simulink model "B20_ATMD_Earthquake"  (R2020b)
settings: Solver=ode45  StartTime=0.0  StopTime=40  FixedStep=Ts  MaxStep=Ts  MinStep=0.005  RelTol=1e-2
values from neighbouring files (symbols this model uses):
  DoS_on = 0    [tuneCusum_Detector1.m]    (also in tuneCusum_Detector2.m)
  EI = 0    [tuneCusum_Detector1.m]    (also in tuneCusum_Detector2.m = 1)
  FDI_amp = 1000e5    (= 100000000)    [tuneCusum_Detector1.m]    (also in tuneCusum_Detector2.m)
  FDI_fr = 1/3.5104    (= 0.284867821331)    [tuneCusum_Detector1.m]    (also in tuneCusum_Detector2.m)
  FDIon = 0    [tuneCusum_Detector1.m]    (also in tuneCusum_Detector2.m)
  K_lqr = lqr(A,B,Q,R)    [tuneCusum_Detector1.m]    (also in tuneCusum_Detector2.m)
  MaxF = 2000e3    (= 2000000)    [tuneCusum_Detector1.m]    (also in tuneCusum_Detector2.m)
  nx = length(A)    [tuneCusum_Detector1.m]    (also in tuneCusum_Detector2.m)
  So = So2(nn)    [tuneCusum_Detector1.m]    (also in tuneCusum_Detector2.m)
  Sys_con = ss(A,[E B],C,D)    [tuneCusum_Detector1.m]    (also in tuneCusum_Detector2.m)
  Sys_unc = ss(A_ref,E_ref,C_ref,DD_ref)    [tuneCusum_Detector1.m]    (also in tuneCusum_Detector2.m)
  Ts = 0.01    [tuneCusum_Detector1.m]    (also in tuneCusum_Detector2.m)
  wg2 = wg^2    [tuneCusum_Detector1.m]    (also in tuneCusum_Detector2.m)
  zwg = 2*zg*wg    [tuneCusum_Detector1.m]    (also in tuneCusum_Detector2.m)
undefined symbols (not defined in the file or in its folder): j
libraries: dspindex x2, simulink x1, eeLuenbergerObserver x1
settings Model: Creator=drsoto  LastModifiedBy=ferch
settings SolverCC: AlgebraicLoopSolver=LineSearch
settings DataIOCC: ReturnWorkspaceOutputs=off
settings DebuggingCC: AlgebraicLoopMsg=none  ArithmeticOperatorsInVariantConditions=warning
settings SFSimCC: SimUseLocalCustomCode=off  CustomCodeUndefinedFunction=UseInterfaceOnly
settings RTWCC: RTWUseLocalCustomCode=off
settings CodeAppCC: StateflowObjectComments=on

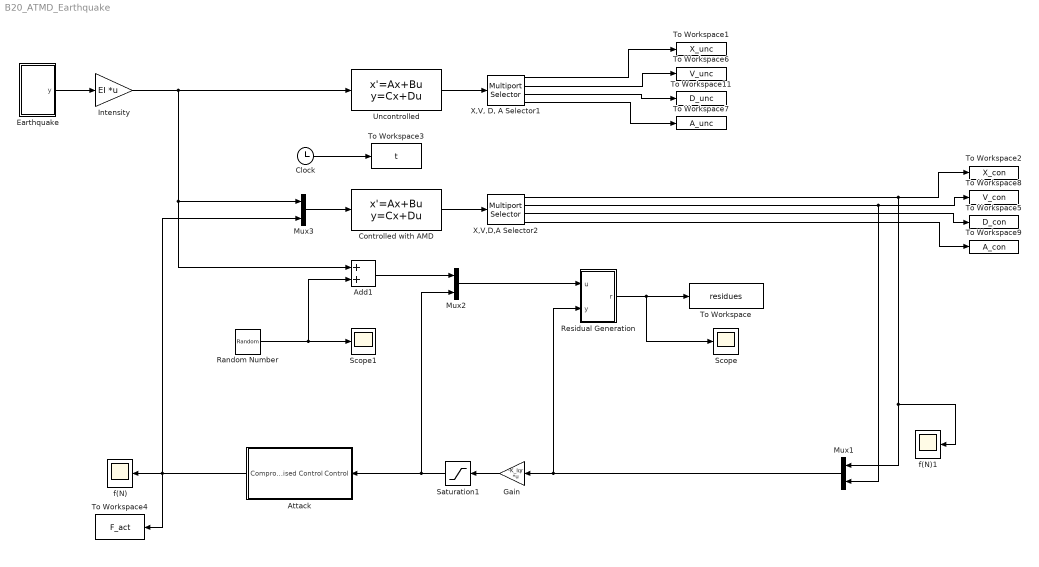
== system B20_ATMD_Earthquake ==
  Add1 : Sum
  Attack : Subsystem
  Clock : Clock
  Controlled with AMD : StateSpace  A=Sys_con.A  B=Sys_con.B  C=Sys_con.C  D=Sys_con.D  InitialCondition=0
  Earthquake : Subsystem
  Gain : Gain  Gain=-K_lqr  Multiplication=Matrix(K*u)
  Intensity : Gain  Gain=EI  Multiplication=Matrix(K*u)
  Mux1 : Mux  Inputs=2
  Mux2 : Mux  Inputs=2
  Mux3 : Mux  Inputs=2
  Random Number : RandomNumber  Variance=0.01  Seed=j  SampleTime=Ts
  "Residual Generation " : Subsystem
  Saturation1 : Saturate  UpperLimit=MaxF  LowerLimit=-MaxF
  Scope : Scope
  Scope1 : Scope
  To Workspace : ToWorkspace  VariableName=residues  SaveFormat=Timeseries  SampleTime=-1
  To Workspace1 : ToWorkspace  VariableName=X_unc  SampleTime=-1
  To Workspace11 : ToWorkspace  VariableName=D_unc  SampleTime=-1
  To Workspace2 : ToWorkspace  VariableName=X_con  SampleTime=-1
  To Workspace3 : ToWorkspace  VariableName=t  SampleTime=-1
      settings: Save2DSignal=2-D array (concatenate along first dimension)
  To Workspace4 : ToWorkspace  VariableName=F_act  SampleTime=-1
  To Workspace5 : ToWorkspace  VariableName=D_con  SampleTime=-1
  To Workspace6 : ToWorkspace  VariableName=V_unc  SampleTime=-1
  To Workspace7 : ToWorkspace  VariableName=A_unc  SampleTime=-1
  To Workspace8 : ToWorkspace  VariableName=V_con  SampleTime=-1
  To Workspace9 : ToWorkspace  VariableName=A_con  SampleTime=-1
  Uncontrolled : StateSpace  A=Sys_unc.A  B=Sys_unc.B  C=Sys_unc.C  D=Sys_unc.D  InitialCondition=0
  "X,V, D, A Selector1" : dspindex/Multiport Selector  rowsOrCols=Rows  idxCellArray={ 1:n,n+1:2*n,2*n+1:3*n,3*n+1:4*n}  idxErrMode=Clip Index
  X,V,D,A Selector2 : dspindex/Multiport Selector  rowsOrCols=Rows  idxCellArray={ 1:n_amd,n_amd+1:2*n_amd,2*n_amd+1:3*n_amd,3*n_amd+1:4*n_amd}  idxErrMode=Clip Index
  f(N) : Scope
  f(N)1 : Scope
  wires:
  Intensity/1 -> Mux3/1, Add1/1, Uncontrolled/1
  Uncontrolled/1 -> "X,V, D, A Selector1"/1
  Controlled with AMD/1 -> X,V,D,A Selector2/1
  Clock/1 -> To Workspace3/1
  "X,V, D, A Selector1"/2 -> To Workspace6/1
  Mux3/1 -> Controlled with AMD/1
  "X,V, D, A Selector1"/4 -> To Workspace7/1
  "X,V, D, A Selector1"/3 -> To Workspace11/1
  X,V,D,A Selector2/3 -> To Workspace5/1
  X,V,D,A Selector2/4 -> To Workspace9/1
  "X,V, D, A Selector1"/1 -> To Workspace1/1
  X,V,D,A Selector2/1 -> Mux1/1, f(N)1/1, To Workspace2/1
  X,V,D,A Selector2/2 -> To Workspace8/1, Mux1/2
  Gain/1 -> Saturation1/1
  Mux1/1 -> "Residual Generation "/2(y), Gain/1
  Random Number/1 -> Scope1/1, Add1/2
  Add1/1 -> Mux2/1
  Saturation1/1 -> Mux2/2, Attack/1(Control)
  "Residual Generation "/1(r) -> Scope/1, To Workspace/1
  Mux2/1 -> "Residual Generation "/1(u)
  Earthquake/1(y) -> Intensity/1
  Attack/1(Compromised Control) -> Mux3/2, f(N)/1, To Workspace4/1

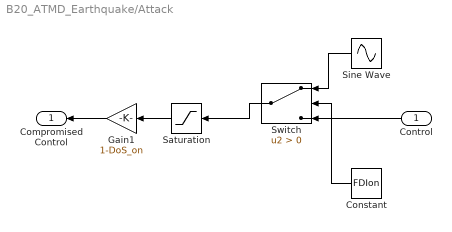
== system B20_ATMD_Earthquake/Attack ==
  Control : Inport
  Constant : Constant  Value=FDIon
  Gain1 : Gain  Gain=1-DoS_on
  Saturation : Saturate  UpperLimit=MaxF  LowerLimit=-MaxF
  Sine Wave : Sin  Amplitude=FDI_amp  Frequency=FDI_fr*2*pi  SampleTime=0
  Switch : Switch  Criteria=u2 > Threshold
  Compromised Control : Outport
  wires:
  Saturation/1 -> Gain1/1
  Switch/1 -> Saturation/1
  Gain1/1 -> Compromised Control/1
  Sine Wave/1 -> Switch/1
  Control/1 -> Switch/3
  Constant/1 -> Switch/2

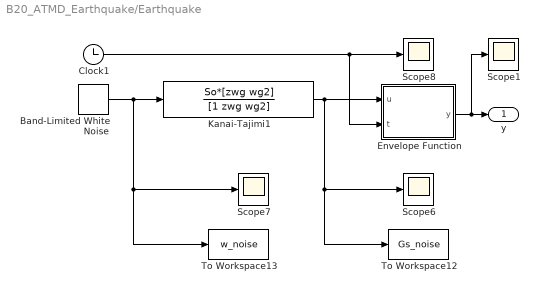
== system B20_ATMD_Earthquake/Earthquake ==
  Band-Limited White Noise : simulink/Sources/Band-Limited White Noise  Cov=[0.1]  Ts=Ts  seed=100
  Clock1 : Clock
  Envelope Function : MATLAB Function  TreatAsAtomicUnit=on
  Kanai-Tajimi1 : TransferFcn  Numerator=So*[zwg wg2]  Denominator=[1 zwg wg2]
  Scope{1,6..8} (4 alike) : Scope
  To Workspace12 : ToWorkspace  VariableName=Gs_noise  SampleTime=-1
  To Workspace13 : ToWorkspace  VariableName=w_noise  SampleTime=-1
  y : Outport
  wires:
  Clock1/1 -> Scope8/1, Envelope Function/2(t)
  Kanai-Tajimi1/1 -> To Workspace12/1, Scope6/1, Envelope Function/1(u)
  Band-Limited White Noise/1 -> Kanai-Tajimi1/1, Scope7/1, To Workspace13/1
  Envelope Function/1(y) -> Scope1/1, y/1

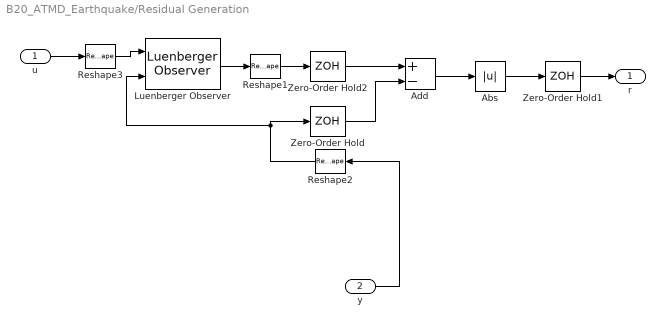
== system B20_ATMD_Earthquake/Residual Generation  ==
  u : Inport
  y : Inport  Port=2
  Abs : Abs
  Add : Sum  Inputs=+-
  Luenberger Observer : eeLuenbergerObserver/Luenberger Observer  StateSpaceType=Continuous-time  Ad=Sys_con.A  Bd=Sys_con.B  Cd=Sys_con.C  Dd=Sys_con.D  A=Sys_con.A  B=Sys_con.B  C=eye(42)  D=Sys_con.B*0  ObserverDesign=Desired eigenvalues  Ld=1  DesiredEigenvalues=[-1:-1:-nx]/5-15  x0=zeros(nx,1)  Tsd=0.1  Ts=Ts
      settings: SourceProductBaseCode=PS
  Reshape1 : Reshape
  Reshape2 : Reshape
  Reshape3 : Reshape
  Zero-Order Hold : ZeroOrderHold  SampleTime=Ts
  Zero-Order Hold1 : ZeroOrderHold  SampleTime=Ts
  Zero-Order Hold2 : ZeroOrderHold  SampleTime=Ts
  r : Outport
  wires:
  Add/1 -> Abs/1
  Luenberger Observer/1 -> Reshape1/1
  Reshape2/1 -> Zero-Order Hold/1, Luenberger Observer/2
  Reshape1/1 -> Zero-Order Hold2/1
  Zero-Order Hold2/1 -> Add/1
  Reshape3/1 -> Luenberger Observer/1
  Abs/1 -> Zero-Order Hold1/1
  Zero-Order Hold/1 -> Add/2
  y/1 -> Reshape2/1
  Zero-Order Hold1/1 -> r/1
  u/1 -> Reshape3/1

== matlab function B20_ATMD_Earthquake/Earthquake/Envelope Function ==
  data: u input; y output; t input
function y = fcn(u,t)
%#codegen
t1=6; % 3seconds
t2 =15;
gam=0.26;
if t <= t1
    a = (t/t1)^2; 
    y=a*u;
elseif t >= t1 && t <= t2
    a = 1 ;
    y=a*u;
elseif t > t2
    a = exp(-gam.*(t-t2));
    y= a*u;
else
    y=0*u;
end
end
